simulink model "Capsuleuse_fermeture_geometrique"  (R2019b)
settings: Solver=VariableStepAuto  StartTime=0.0  StopTime=10.0  RelTol=1e-3
PreLoadFcn:
  | addpath('Simscape')
model workspace (MATLAB code in the model file):
  | % Simscape(TM) Multibody(TM) version: 7.0
  | 
  | % This is a model data file derived from a Simscape Multibody Import XML file using the smimport function.
  | % The data in this file sets the block parameter values in an imported Simscape Multibody model.
  | % For more information on this file, see the smimport function help page in the Simscape Multibody documentation.
  | % You can modify numerical values, but avoid any other changes to this file.
  | % Do not add code to this file. Do not edit the physical units shown in comments.
  | 
  | %%%VariableName:smiData
  | 
  | 
  | %============= RigidTransform =============%
  | 
  | %Initialize the RigidTransform structure array by filling in null values.
  | smiData.RigidTransform(76).translation = [0.0 0.0 0.0];
  | smiData.RigidTransform(76).angle = 0.0;
  | smiData.RigidTransform(76).axis = [0.0 0.0 0.0];
  | smiData.RigidTransform(76).ID = '';
  | 
  | %Translation Method - Cartesian
  | %Rotation Method - Arbitrary Axis
  | smiData.RigidTransform(1).translation = [0 0 0];  % mm
  | smiData.RigidTransform(1).angle = 2.2204460492503136e-16;  % rad
  | smiData.RigidTransform(1).axis = [-1 0 -0];
  | smiData.RigidTransform(1).ID = 'B[Bati-1:-:]';
  | 
  | %Translation Method - Cartesian
  | %Rotation Method - Arbitrary Axis
  | smiData.RigidTransform(2).translation = [0 0 0];  % mm
  | smiData.RigidTransform(2).angle = 3.1415926535897931;  % rad
  | smiData.RigidTransform(2).axis = [0 -1 -5.5511151231257839e-17];
  | smiData.RigidTransform(2).ID = 'F[Bati-1:-:]';
  | 
  | %Translation Method - Cartesian
  | %Rotation Method - Arbitrary Axis
  | smiData.RigidTransform(3).translation = [-1.4210854715202004e-14 8.8817841970012523e-14 125];  % mm
  | smiData.RigidTransform(3).angle = 2.0943951023931953;  % rad
  | smiData.RigidTransform(3).axis = [-0.57735026918962584 -0.57735026918962584 -0.57735026918962584];
  | smiData.RigidTransform(3).ID = 'B[Bati-1:-:Croix_de_Malte-1]';
  | 
  | %Translation Method - Cartesian
  | %Rotation Method - Arbitrary Axis
  | smiData.RigidTransform(4).translation = [1.8690460720473507e-12 22.000000000000014 -2.2892209790695388e-28];  % mm
  | smiData.RigidTransform(4).angle = 2.0943951023931953;  % rad
  | smiData.RigidTransform(4).axis = [-0.57735026918962584 -0.57735026918962562 -0.57735026918962595];
  | smiData.RigidTransform(4).ID = 'F[Bati-1:-:Croix_de_Malte-1]';
  | 
  | %Translation Method - Cartesian
  | %Rotation Method - Arbitrary Axis
  | smiData.RigidTransform(5).translation = [0 4.6185277824406512e-14 -3.5527136788005009e-15];  % mm
  | smiData.RigidTransform(5).angle = 2.0943951023931953;  % rad
  | smiData.RigidTransform(5).axis = [-0.57735026918962584 -0.57735026918962584 -0.57735026918962584];
  | smiData.RigidTransform(5).ID = 'B[Bati-1:-:Moteur-1]';
  | 
  | %Translation Method - Cartesian
  | %Rotation Method - Arbitrary Axis
  | smiData.RigidTransform(6).translation = [2.3777209295873426e-14 24.999999999999876 -3.6840445277123552e-15];  % mm
  | smiData.RigidTransform(6).angle = 2.0943951023931962;  % rad
  | smiData.RigidTransform(6).axis = [-0.57735026918962595 -0.57735026918962529 -0.57735026918962606];
  | smiData.RigidTransform(6).ID = 'F[Bati-1:-:Moteur-1]';
  | 
  | %Translation Method - Cartesian
  | %Rotation Method - Arbitrary Axis
  | smiData.RigidTransform(7).translation = [-18.73832970144344 11 -32.173358543987945];  % mm
  | smiData.RigidTransform(7).angle = 1.7177715174584023;  % rad
  | smiData.RigidTransform(7).axis = [-0.35740674433659403 -0.35740674433659386 0.86285620946101627];
  | smiData.RigidTransform(7).ID = 'B[Croix_de_Malte-1:-:rouleau galet-1]';
  | 
  | %Translation Method - Cartesian
  | %Rotation Method - Arbitrary Axis
  | smiData.RigidTransform(8).translation = [29.594858329028312 1.0000000000000657 -43.752922275812764];  % mm
  | smiData.RigidTransform(8).angle = 1.7206562415507236;  % rad
  | smiData.RigidTransform(8).axis = [0.36042318328087997 0.36042318328088008 0.86034310475958042];
  | smiData.RigidTransform(8).ID = 'F[Croix_de_Malte-1:-:rouleau galet-1]';
  | 
  | %Translation Method - Cartesian
  | %Rotation Method - Arbitrary Axis
  | smiData.RigidTransform(9).translation = [0 12.574722564734881 -0.13414733414733593];  % mm
  | smiData.RigidTransform(9).angle = 2.0943951023931953;  % rad
  | smiData.RigidTransform(9).axis = [-0.57735026918962584 -0.57735026918962584 -0.57735026918962584];
  | smiData.RigidTransform(9).ID = 'B[rouleau galet-1:-:Moteur-1]';
  | 
  | %Translation Method - Cartesian
  | %Rotation Method - Arbitrary Axis
  | smiData.RigidTransform(10).translation = [-4.2632564145606011e-14 25.574722564734707 88.390000000000057];  % mm
  | smiData.RigidTransform(10).angle = 2.0943951023931966;  % rad
  | smiData.RigidTransform(10).axis = [-0.57735026918962606 -0.5773502691896254 -0.57735026918962573];
  | smiData.RigidTransform(10).ID = 'F[rouleau galet-1:-:Moteur-1]';
  | 
  | %Translation Method - Cartesian
  | %Rotation Method - Arbitrary Axis
  | smiData.RigidTransform(11).translation = [-0.35889856916805629 20.000000000000071 84.999999999999986];  % mm
  | smiData.RigidTransform(11).angle = 3.1415926535897931;  % rad
  | smiData.RigidTransform(11).axis = [0 -0.70710678118654746 0.70710678118654757];
  | smiData.RigidTransform(11).ID = 'AssemblyGround[Bati-1:vis M6x20-2]';
  | 
  | %Translation Method - Cartesian
  | %Rotation Method - Arbitrary Axis
  | smiData.RigidTransform(12).translation = [0 7.0000000000000862 125];  % mm
  | smiData.RigidTransform(12).angle = 2.0943951023931957;  % rad
  | smiData.RigidTransform(12).axis = [-0.57735026918962562 -0.57735026918962562 0.57735026918962595];
  | smiData.RigidTransform(12).ID = 'AssemblyGround[Bati-1:boitier-1]';
  | 
  | %Translation Method - Cartesian
  | %Rotation Method - Arbitrary Axis
  | smiData.RigidTransform(13).translation = [69.999999999999986 12.000000000000032 -30.000000000000025];  % mm
  | smiData.RigidTransform(13).angle = 3.1415926535897931;  % rad
  | smiData.RigidTransform(13).axis = [0 -0.70710678118654746 0.70710678118654757];
  | smiData.RigidTransform(13).ID = 'AssemblyGround[Bati-1:plaque de base-1]';
  | 
  | %Translation Method - Cartesian
  | %Rotation Method - Arbitrary Axis
  | smiData.RigidTransform(14).translation = [39.999999999999993 20.000000000000089 125];  % mm
  | smiData.RigidTransform(14).angle = 3.1415926535897931;  % rad
  | smiData.RigidTransform(14).axis = [0 -0.70710678118654746 0.70710678118654757];
  | smiData.RigidTransform(14).ID = 'AssemblyGround[Bati-1:vis M6x20-1]';
  | 
  | %Translation Method - Cartesian
  | %Rotation Method - Arbitrary Axis
  | smiData.RigidTransform(15).translation = [194.99999999999994 25.000000000000124 235];  % mm
  | smiData.RigidTransform(15).angle = 3.1415926535897931;  % rad
  | smiData.RigidTransform(15).axis = [0 -0.70710678118654746 0.70710678118654757];
  | smiData.RigidTransform(15).ID = 'AssemblyGround[Bati-1:vis M8x25-2]';
  | 
  | %Translation Method - Cartesian
  | %Rotation Method - Arbitrary Axis
  | smiData.RigidTransform(16).translation = [-120.00000000000001 25.000000000000021 -55.000000000000043];  % mm
  | smiData.RigidTransform(16).angle = 3.1415926535897931;  % rad
  | smiData.RigidTransform(16).axis = [0 -0.70710678118654746 0.70710678118654757];
  | smiData.RigidTransform(16).ID = 'AssemblyGround[Bati-1:vis M8x25-3]';
  | 
  | %Translation Method - Cartesian
  | %Rotation Method - Arbitrary Axis
  | smiData.RigidTransform(17).translation = [194.99999999999994 25.00000000000006 39.999999999999986];  % mm
  | smiData.RigidTransform(17).angle = 3.1415926535897931;  % rad
  | smiData.RigidTransform(17).axis = [0 -0.70710678118654746 0.70710678118654757];
  | smiData.RigidTransform(17).ID = 'AssemblyGround[Bati-1:vis M8x25-1]';
  | 
  | %Translation Method - Cartesian
  | %Rotation Method - Arbitrary Axis
  | smiData.RigidTransform(18).translation = [-0.35889856916804241 20.000000000000099 165];  % mm
  | smiData.RigidTransform(18).angle = 3.1415926535897931;  % rad
  | smiData.RigidTransform(18).axis = [0 -0.70710678118654746 0.70710678118654757];
  | smiData.RigidTransform(18).ID = 'AssemblyGround[Bati-1:vis M6x20-3]';
  | 
  | %Translation Method - Cartesian
  | %Rotation Method - Arbitrary Axis
  | smiData.RigidTransform(19).translation = [-10.999999999999829 224.64380550980667 146.35619449019265];  % mm
  | smiData.RigidTransform(19).angle = 3.1415926535897833;  % rad
  | smiData.RigidTransform(19).axis = [0.70710678118654768 -2.3482086884408253e-15 0.70710678118654735];
  | smiData.RigidTransform(19).ID = 'AssemblyGround[Bati-1:rampe-1]';
  | 
  | %Translation Method - Cartesian
  | %Rotation Method - Arbitrary Axis
  | smiData.RigidTransform(20).translation = [-120.00000000000006 296.00000000000006 -54.999999999999929];  % mm
  | smiData.RigidTransform(20).angle = 1.6089415660457551;  % rad
  | smiData.RigidTransform(20).axis = [-0.96256421976262596 -0.19166392831303336 -0.19166392831303336];
  | smiData.RigidTransform(20).ID = 'AssemblyGround[Bati-1:vis M8x20-3]';
  | 
  | %Translation Method - Cartesian
  | %Rotation Method - Arbitrary Axis
  | smiData.RigidTransform(21).translation = [-109.00000000000003 310 -44.000000000000028];  % mm
  | smiData.RigidTransform(21).angle = 3.1415926535897931;  % rad
  | smiData.RigidTransform(21).axis = [0 -0.70710678118654746 0.70710678118654757];
  | smiData.RigidTransform(21).ID = 'AssemblyGround[Bati-1:pied-3]';
  | 
  | %Translation Method - Cartesian
  | %Rotation Method - Arbitrary Axis
  | smiData.RigidTransform(22).translation = [0 1.9999999999999658 -42.499999999999986];  % mm
  | smiData.RigidTransform(22).angle = 1.6654317068748059;  % rad
  | smiData.RigidTransform(22).axis = [-0.90957578911615289 -0.29382978393427672 -0.29382978393427672];
  | smiData.RigidTransform(22).ID = 'AssemblyGround[Bati-1:vis M6x20-6]';
  | 
  | %Translation Method - Cartesian
  | %Rotation Method - Arbitrary Axis
  | smiData.RigidTransform(23).translation = [205.99999999999997 310.00000000000011 246];  % mm
  | smiData.RigidTransform(23).angle = 3.1415926535897931;  % rad
  | smiData.RigidTransform(23).axis = [0 -0.70710678118654746 0.70710678118654757];
  | smiData.RigidTransform(23).ID = 'AssemblyGround[Bati-1:pied-1]';
  | 
  | %Translation Method - Cartesian
  | %Rotation Method - Arbitrary Axis
  | smiData.RigidTransform(24).translation = [194.99999999999994 296.00000000000011 235.00000000000003];  % mm
  | smiData.RigidTransform(24).angle = 1.6089415660457551;  % rad
  | smiData.RigidTransform(24).axis = [-0.96256421976262596 -0.19166392831303336 -0.19166392831303336];
  | smiData.RigidTransform(24).ID = 'AssemblyGround[Bati-1:vis M8x20-2]';
  | 
  | %Translation Method - Cartesian
  | %Rotation Method - Arbitrary Axis
  | smiData.RigidTransform(25).translation = [-32.000000000000071 185.00000000000009 418.00000000000006];  % mm
  | smiData.RigidTransform(25).angle = 1.5707963267948968;  % rad
  | smiData.RigidTransform(25).axis = [-1 2.081668171172168e-16 2.081668171172168e-16];
  | smiData.RigidTransform(25).ID = 'AssemblyGround[Bati-1:support-1]';
  | 
  | %Translation Method - Cartesian
  | %Rotation Method - Arbitrary Axis
  | smiData.RigidTransform(26).translation = [205.99999999999997 310.00000000000006 51.000000000000028];  % mm
  | smiData.RigidTransform(26).angle = 3.1415926535897931;  % rad
  | smiData.RigidTransform(26).axis = [0 -0.70710678118654746 0.70710678118654757];
  | smiData.RigidTransform(26).ID = 'AssemblyGround[Bati-1:pied-2]';
  | 
  | %Translation Method - Cartesian
  | %Rotation Method - Arbitrary Axis
  | smiData.RigidTransform(27).translation = [0 7.0000000000000409 0];  % mm
  | smiData.RigidTransform(27).angle = 3.1415926535897931;  % rad
  | smiData.RigidTransform(27).axis = [0.70710678118654768 1.218024257459634e-16 0.70710678118654735];
  | smiData.RigidTransform(27).ID = 'AssemblyGround[Bati-1:motoreducteur-1]';
  | 
  | %Translation Method - Cartesian
  | %Rotation Method - Arbitrary Axis
  | smiData.RigidTransform(28).translation = [42.499999999999993 2.0000000000001523 0];  % mm
  | smiData.RigidTransform(28).angle = 1.7612805946572963;  % rad
  | smiData.RigidTransform(28).axis = [-0.82559845262457221 -0.39899072359135895 -0.39899072359135845];
  | smiData.RigidTransform(28).ID = 'AssemblyGround[Bati-1:vis M6x20-5]';
  | 
  | %Translation Method - Cartesian
  | %Rotation Method - Arbitrary Axis
  | smiData.RigidTransform(29).translation = [299.99999999999994 316.00000000000017 430];  % mm
  | smiData.RigidTransform(29).angle = 3.1415926535897931;  % rad
  | smiData.RigidTransform(29).axis = [0 -0.70710678118654746 0.70710678118654757];
  | smiData.RigidTransform(29).ID = 'AssemblyGround[Bati-1:bati-1]';
  | 
  | %Translation Method - Cartesian
  | %Rotation Method - Arbitrary Axis
  | smiData.RigidTransform(30).translation = [194.99999999999991 296.00000000000006 40.000000000000043];  % mm
  | smiData.RigidTransform(30).angle = 1.6089415660457551;  % rad
  | smiData.RigidTransform(30).axis = [-0.96256421976262596 -0.19166392831303336 -0.19166392831303336];
  | smiData.RigidTransform(30).ID = 'AssemblyGround[Bati-1:vis M8x20-1]';
  | 
  | %Translation Method - Cartesian
  | %Rotation Method - Arbitrary Axis
  | smiData.RigidTransform(31).translation = [-40.000000000000007 20.000000000000089 125.00000000000003];  % mm
  | smiData.RigidTransform(31).angle = 3.1415926535897931;  % rad
  | smiData.RigidTransform(31).axis = [0 -0.70710678118654746 0.70710678118654757];
  | smiData.RigidTransform(31).ID = 'AssemblyGround[Bati-1:vis M6x20-4]';
  | 
  | %Translation Method - Cartesian
  | %Rotation Method - Arbitrary Axis
  | smiData.RigidTransform(32).translation = [0 2.0000000000000751 42.500000000000007];  % mm
  | smiData.RigidTransform(32).angle = 1.6333821857835207;  % rad
  | smiData.RigidTransform(32).axis = [-0.9392939931105766 -0.24261780077561093 -0.24261780077561074];
  | smiData.RigidTransform(32).ID = 'AssemblyGround[Bati-1:vis M6x20-7]';
  | 
  | %Translation Method - Cartesian
  | %Rotation Method - Arbitrary Axis
  | smiData.RigidTransform(33).translation = [-42.500000000000007 2.000000000000107 0];  % mm
  | smiData.RigidTransform(33).angle = 1.7546548549139718;  % rad
  | smiData.RigidTransform(33).axis = [-0.83118471645013647 -0.3931488058863376 -0.39314880588633738];
  | smiData.RigidTransform(33).ID = 'AssemblyGround[Bati-1:vis M6x20-8]';
  | 
  | %Translation Method - Cartesian
  | %Rotation Method - Arbitrary Axis
  | smiData.RigidTransform(34).translation = [-35.355339059327292 213.50000000000003 -35.355339059327434];  % mm
  | smiData.RigidTransform(34).angle = 3.1415926535897909;  % rad
  | smiData.RigidTransform(34).axis = [1.2601194582917002e-15 0.70710678118654746 -0.70710678118654757];
  | smiData.RigidTransform(34).ID = 'AssemblyGround[Croix_de_Malte-1:ecrou M12-1]';
  | 
  | %Translation Method - Cartesian
  | %Rotation Method - Arbitrary Axis
  | smiData.RigidTransform(35).translation = [-15.999999999999963 16.999999999999996 6.9999999999999503];  % mm
  | smiData.RigidTransform(35).angle = 2.0943951023931953;  % rad
  | smiData.RigidTransform(35).axis = [0.57735026918962584 -0.57735026918962584 0.57735026918962584];
  | smiData.RigidTransform(35).ID = 'AssemblyGround[Croix_de_Malte-1:goupille D6-1]';
  | 
  | %Translation Method - Cartesian
  | %Rotation Method - Arbitrary Axis
  | smiData.RigidTransform(36).translation = [15.999999999999993 16.999999999999993 7.0000000000000338];  % mm
  | smiData.RigidTransform(36).angle = 3.0512029265937719;  % rad
  | smiData.RigidTransform(36).axis = [0.045225659969685389 0.70638326695934206 -0.70638326695934206];
  | smiData.RigidTransform(36).ID = 'AssemblyGround[Croix_de_Malte-1:goupille D6-2]';
  | 
  | %Translation Method - Cartesian
  | %Rotation Method - Arbitrary Axis
  | smiData.RigidTransform(37).translation = [0 180 0];  % mm
  | smiData.RigidTransform(37).angle = 1.5707963267948966;  % rad
  | smiData.RigidTransform(37).axis = [0 0 1];
  | smiData.RigidTransform(37).ID = 'AssemblyGround[Croix_de_Malte-1:bride-1]';
  | 
  | %Translation Method - Cartesian
  | %Rotation Method - Arbitrary Axis
  | smiData.RigidTransform(38).translation = [67.500000000000028 209.99999999999997 0];  % mm
  | smiData.RigidTransform(38).angle = 2.0943951023931953;  % rad
  | smiData.RigidTransform(38).axis = [0.57735026918962584 -0.57735026918962584 0.57735026918962584];
  | smiData.RigidTransform(38).ID = 'AssemblyGround[Croix_de_Malte-1:vis M6x30-2]';
  | 
  | %Translation Method - Cartesian
  | %Rotation Method - Arbitrary Axis
  | smiData.RigidTransform(39).translation = [0 221 0];  % mm
  | smiData.RigidTransform(39).angle = 3.1415926535897922;  % rad
  | smiData.RigidTransform(39).axis = [6.713347862852846e-16 0.70710678118654746 -0.70710678118654757];
  | smiData.RigidTransform(39).ID = 'AssemblyGround[Croix_de_Malte-1:plateau-1]';
  | 
  | %Translation Method - Cartesian
  | %Rotation Method - Arbitrary Axis
  | smiData.RigidTransform(40).translation = [0 210 -67.5];  % mm
  | smiData.RigidTransform(40).angle = 2.0943951023931953;  % rad
  | smiData.RigidTransform(40).axis = [0.57735026918962584 -0.57735026918962584 0.57735026918962584];
  | smiData.RigidTransform(40).ID = 'AssemblyGround[Croix_de_Malte-1:vis M6x30-4]';
  | 
  | %Translation Method - Cartesian
  | %Rotation Method - Arbitrary Axis
  | smiData.RigidTransform(41).translation = [-35.355339059327292 195 -35.355339059327434];  % mm
  | smiData.RigidTransform(41).angle = 1.5744668381809315;  % rad
  | smiData.RigidTransform(41).axis = [-0.9963362084947659 0.060473794499247502 0.06047379449924746];
  | smiData.RigidTransform(41).ID = 'AssemblyGround[Croix_de_Malte-1:vis a billes-1]';
  | 
  | %Translation Method - Cartesian
  | %Rotation Method - Arbitrary Axis
  | smiData.RigidTransform(42).translation = [0 145 0];  % mm
  | smiData.RigidTransform(42).angle = 1.7177715174584023;  % rad
  | smiData.RigidTransform(42).axis = [-0.35740674433659392 -0.35740674433659392 0.86285620946101627];
  | smiData.RigidTransform(42).ID = 'AssemblyGround[Croix_de_Malte-1:limiteur couple-1]';
  | 
  | %Translation Method - Cartesian
  | %Rotation Method - Arbitrary Axis
  | smiData.RigidTransform(43).translation = [0 159.99999999999994 -22.500000000000007];  % mm
  | smiData.RigidTransform(43).angle = 1.8369463418012444;  % rad
  | smiData.RigidTransform(43).axis = [-3.8857805861880479e-16 -3.0765813436776594e-16 1];
  | smiData.RigidTransform(43).ID = 'AssemblyGround[Croix_de_Malte-1:mecanindus-1]';
  | 
  | %Translation Method - Cartesian
  | %Rotation Method - Arbitrary Axis
  | smiData.RigidTransform(44).translation = [0 210.00000000000003 67.5];  % mm
  | smiData.RigidTransform(44).angle = 2.0943951023931953;  % rad
  | smiData.RigidTransform(44).axis = [0.57735026918962584 -0.57735026918962584 0.57735026918962584];
  | smiData.RigidTransform(44).ID = 'AssemblyGround[Croix_de_Malte-1:vis M6x30-1]';
  | 
  | %Translation Method - Cartesian
  | %Rotation Method - Arbitrary Axis
  | smiData.RigidTransform(45).translation = [-67.499999999999972 210 0];  % mm
  | smiData.RigidTransform(45).angle = 2.0943951023931953;  % rad
  | smiData.RigidTransform(45).axis = [0.57735026918962584 -0.57735026918962584 0.57735026918962584];
  | smiData.RigidTransform(45).ID = 'AssemblyGround[Croix_de_Malte-1:vis M6x30-3]';
  | 
  | %Translation Method - Cartesian
  | %Rotation Method - Arbitrary Axis
  | smiData.RigidTransform(46).translation = [0 0 0];  % mm
  | smiData.RigidTransform(46).angle = 0;  % rad
  | smiData.RigidTransform(46).axis = [0 0 0];
  | smiData.RigidTransform(46).ID = 'AssemblyGround[Croix_de_Malte-1:6004-2:BI 6004-1]';
  | 
  | %Translation Method - Cartesian
  | %Rotation Method - Arbitrary Axis
  | smiData.RigidTransform(47).translation = [0 0 0];  % mm
  | smiData.RigidTransform(47).angle = 0;  % rad
  | smiData.RigidTransform(47).axis = [0 0 0];
  | smiData.RigidTransform(47).ID = 'AssemblyGround[Croix_de_Malte-1:6004-2:bille 6004-1]';
  | 
  | %Translation Method - Cartesian
  | %Rotation Method - Arbitrary Axis
  | smiData.RigidTransform(48).translation = [0 0 0];  % mm
  | smiData.RigidTransform(48).angle = 0;  % rad
  | smiData.RigidTransform(48).axis = [0 0 0];
  | smiData.RigidTransform(48).ID = 'AssemblyGround[Croix_de_Malte-1:6004-2:BE 6004-1]';
  | 
  | %Translation Method - Cartesian
  | %Rotation Method - Arbitrary Axis
  | smiData.RigidTransform(49).translation = [87.500000000000014 134 0];  % mm
  | smiData.RigidTransform(49).angle = 1.5707963267948966;  % rad
  | smiData.RigidTransform(49).axis = [0 0 1];
  | smiData.RigidTransform(49).ID = 'AssemblyGround[Croix_de_Malte-1:6004-2]';
  | 
  | %Translation Method - Cartesian
  | %Rotation Method - Arbitrary Axis
  | smiData.RigidTransform(50).translation = [0 -19 49.999999999999986];  % mm
  | smiData.RigidTransform(50).angle = 1.5707963267948966;  % rad
  | smiData.RigidTransform(50).axis = [0 0 1];
  | smiData.RigidTransform(50).ID = 'AssemblyGround[Croix_de_Malte-1:doigt-1]';
  | 
  | %Translation Method - Cartesian
  | %Rotation Method - Arbitrary Axis
  | smiData.RigidTransform(51).translation = [0 -1.0000000000000009 0];  % mm
  | smiData.RigidTransform(51).angle = 1.5707963267948966;  % rad
  | smiData.RigidTransform(51).axis = [0 0 1];
  | smiData.RigidTransform(51).ID = 'AssemblyGround[Croix_de_Malte-1:axe de sortie-1]';
  | 
  | %Translation Method - Cartesian
  | %Rotation Method - Arbitrary Axis
  | smiData.RigidTransform(52).translation = [0 0 0];  % mm
  | smiData.RigidTransform(52).angle = 2.0943951023931966;  % rad
  | smiData.RigidTransform(52).axis = [-0.57735026918962618 -0.57735026918962606 0.57735026918962495];
  | smiData.RigidTransform(52).ID = 'AssemblyGround[Croix_de_Malte-1:croix-1]';
  | 
  | %Translation Method - Cartesian
  | %Rotation Method - Arbitrary Axis
  | smiData.RigidTransform(53).translation = [0 -1.0000000000000009 0];  % mm
  | smiData.RigidTransform(53).angle = 2.0943951023931966;  % rad
  | smiData.RigidTransform(53).axis = [0.57735026918962495 -0.57735026918962618 0.57735026918962618];
  | smiData.RigidTransform(53).ID = 'AssemblyGround[Croix_de_Malte-1:capteur-1]';
  | 
  | %Translation Method - Cartesian
  | %Rotation Method - Arbitrary Axis
  | smiData.RigidTransform(54).translation = [0 11.999999999999998 16.000000000000014];  % mm
  | smiData.RigidTransform(54).angle = 2.0943951023931953;  % rad
  | smiData.RigidTransform(54).axis = [0.57735026918962584 -0.57735026918962584 0.57735026918962584];
  | smiData.RigidTransform(54).ID = 'AssemblyGround[Croix_de_Malte-1:vis M6x25-1]';
  | 
  | %Translation Method - Cartesian
  | %Rotation Method - Arbitrary Axis
  | smiData.RigidTransform(55).translation = [0 0 0];  % mm
  | smiData.RigidTransform(55).angle = 0;  % rad
  | smiData.RigidTransform(55).axis = [0 0 0];
  | smiData.RigidTransform(55).ID = 'AssemblyGround[Croix_de_Malte-1:6004-1:BI 6004-1]';
  | 
  | %Translation Method - Cartesian
  | %Rotation Method - Arbitrary Axis
  | smiData.RigidTransform(56).translation = [0 0 0];  % mm
  | smiData.RigidTransform(56).angle = 0;  % rad
  | smiData.RigidTransform(56).axis = [0 0 0];
  | smiData.RigidTransform(56).ID = 'AssemblyGround[Croix_de_Malte-1:6004-1:bille 6004-1]';
  | 
  | %Translation Method - Cartesian
  | %Rotation Method - Arbitrary Axis
  | smiData.RigidTransform(57).translation = [0 0 0];  % mm
  | smiData.RigidTransform(57).angle = 0;  % rad
  | smiData.RigidTransform(57).axis = [0 0 0];
  | smiData.RigidTransform(57).ID = 'AssemblyGround[Croix_de_Malte-1:6004-1:BE 6004-1]';
  | 
  | %Translation Method - Cartesian
  | %Rotation Method - Arbitrary Axis
  | smiData.RigidTransform(58).translation = [87.500000000000014 55.999999999999979 0];  % mm
  | smiData.RigidTransform(58).angle = 1.5707963267948966;  % rad
  | smiData.RigidTransform(58).axis = [0 0 1];
  | smiData.RigidTransform(58).ID = 'AssemblyGround[Croix_de_Malte-1:6004-1]';
  | 
  | %Translation Method - Cartesian
  | %Rotation Method - Arbitrary Axis
  | smiData.RigidTransform(59).translation = [0 -12.000000000000004 0];  % mm
  | smiData.RigidTransform(59).angle = 2.0943951023931948;  % rad
  | smiData.RigidTransform(59).axis = [0.57735026918962629 0.57735026918962562 0.57735026918962551];
  | smiData.RigidTransform(59).ID = 'AssemblyGround[Moteur-1:indexeur-1]';
  | 
  | %Translation Method - Cartesian
  | %Rotation Method - Arbitrary Axis
  | smiData.RigidTransform(60).translation = [0 -24.000000000000007 0];  % mm
  | smiData.RigidTransform(60).angle = 2.0943951023931953;  % rad
  | smiData.RigidTransform(60).axis = [-0.57735026918962584 0.57735026918962584 0.57735026918962584];
  | smiData.RigidTransform(60).ID = 'AssemblyGround[Moteur-1:capteur-1]';
  | 
  | %Translation Method - Cartesian
  | %Rotation Method - Arbitrary Axis
  | smiData.RigidTransform(61).translation = [0 -20.499999999999886 88.390000000000001];  % mm
  | smiData.RigidTransform(61).angle = 1.6445462178112022;  % rad
  | smiData.RigidTransform(61).axis = [-0.9288418077937356 0.26196650176545955 0.26196650176545944];
  | smiData.RigidTransform(61).ID = 'AssemblyGround[Moteur-1:ecrou M8-1]';
  | 
  | %Translation Method - Cartesian
  | %Rotation Method - Arbitrary Axis
  | smiData.RigidTransform(62).translation = [0 -13.000000000000005 0];  % mm
  | smiData.RigidTransform(62).angle = 2.0943951023931948;  % rad
  | smiData.RigidTransform(62).axis = [-0.57735026918962618 -0.57735026918962551 0.57735026918962562];
  | smiData.RigidTransform(62).ID = 'AssemblyGround[Moteur-1:arbre moteur-1]';
  | 
  | %Translation Method - Cartesian
  | %Rotation Method - Arbitrary Axis
  | smiData.RigidTransform(63).translation = [0 17 -35.000000000000007];  % mm
  | smiData.RigidTransform(63).angle = 2.0943951023931953;  % rad
  | smiData.RigidTransform(63).axis = [0.57735026918962573 0.57735026918962573 -0.57735026918962584];
  | smiData.RigidTransform(63).ID = 'AssemblyGround[Moteur-1:goupille D10-1]';
  | 
  | %Translation Method - Cartesian
  | %Rotation Method - Arbitrary Axis
  | smiData.RigidTransform(64).translation = [35 0 -35.000000000000014];  % mm
  | smiData.RigidTransform(64).angle = 2.0943951023931948;  % rad
  | smiData.RigidTransform(64).axis = [0.57735026918962562 -0.57735026918962618 0.57735026918962551];
  | smiData.RigidTransform(64).ID = 'AssemblyGround[Moteur-1:maneton-1]';
  | 
  | %Translation Method - Cartesian
  | %Rotation Method - Arbitrary Axis
  | smiData.RigidTransform(65).translation = [0 -30.000000000000021 -50.000000000000014];  % mm
  | smiData.RigidTransform(65).angle = 1.6401005108791142;  % rad
  | smiData.RigidTransform(65).axis = [0.25448752703143285 0.25448752703143285 0.93299099522495466];
  | smiData.RigidTransform(65).ID = 'AssemblyGround[Moteur-1:doigt-1]';
  | 
  | %Translation Method - Cartesian
  | %Rotation Method - Arbitrary Axis
  | smiData.RigidTransform(66).translation = [0 0 88.390000000000001];  % mm
  | smiData.RigidTransform(66).angle = 1.5707963267948966;  % rad
  | smiData.RigidTransform(66).axis = [0 0 1];
  | smiData.RigidTransform(66).ID = 'AssemblyGround[Moteur-1:rondelle galet-1]';
  | 
  | %Translation Method - Cartesian
  | %Rotation Method - Arbitrary Axis
  | smiData.RigidTransform(67).translation = [0 -14.000000000000005 88.390000000000015];  % mm
  | smiData.RigidTransform(67).angle = 1.5707963267948966;  % rad
  | smiData.RigidTransform(67).axis = [0 0 1];
  | smiData.RigidTransform(67).ID = 'AssemblyGround[Moteur-1:rondelle galet-2]';
  | 
  | %Translation Method - Cartesian
  | %Rotation Method - Arbitrary Axis
  | smiData.RigidTransform(68).translation = [0 11.99999999999989 88.390000000000015];  % mm
  | smiData.RigidTransform(68).angle = 2.3824818043914275;  % rad
  | smiData.RigidTransform(68).axis = [-0.64841380796894177 0.64841380796894188 -0.39889731419305452];
  | smiData.RigidTransform(68).ID = 'AssemblyGround[Moteur-1:axe galet-1]';
  | 
  | %Translation Method - Cartesian
  | %Rotation Method - Arbitrary Axis
  | smiData.RigidTransform(69).translation = [0 5.9999999999999876 -16.000000000000011];  % mm
  | smiData.RigidTransform(69).angle = 2.8654427051283657;  % rad
  | smiData.RigidTransform(69).axis = [0.13895917020031051 -0.70024650981537961 0.70024650981537961];
  | smiData.RigidTransform(69).ID = 'AssemblyGround[Moteur-1:vis M6x30-1]';
  | 
  | %Translation Method - Cartesian
  | %Rotation Method - Arbitrary Axis
  | smiData.RigidTransform(70).translation = [16.000000000000036 -24.000000000000014 -7.0000000000000107];  % mm
  | smiData.RigidTransform(70).angle = 2.0943951023931953;  % rad
  | smiData.RigidTransform(70).axis = [-0.57735026918962584 0.57735026918962584 0.57735026918962584];
  | smiData.RigidTransform(70).ID = 'AssemblyGround[Moteur-1:goupille D6-1]';
  | 
  | %Translation Method - Cartesian
  | %Rotation Method - Arbitrary Axis
  | smiData.RigidTransform(71).translation = [3.0000000000001505 143.00000000000006 -6.8543636114536088];  % mm
  | smiData.RigidTransform(71).angle = 3.1415926535897922;  % rad
  | smiData.RigidTransform(71).axis = [-3.3080175810533039e-16 -0.70710678118654746 0.70710678118654757];
  | smiData.RigidTransform(71).ID = 'AssemblyGround[Moteur-1:clavette-1]';
  | 
  | %Translation Method - Cartesian
  | %Rotation Method - Arbitrary Axis
  | smiData.RigidTransform(72).translation = [0.48219033392770183 152.99999999999991 0.1322591466277776];  % mm
  | smiData.RigidTransform(72).angle = 1.5886069344924167;  % rad
  | smiData.RigidTransform(72).axis = [-0.13228012687504107 -0.13228012687504107 0.98234613862316666];
  | smiData.RigidTransform(72).ID = 'AssemblyGround[Moteur-1:rondelle arbre moteur-1]';
  | 
  | %Translation Method - Cartesian
  | %Rotation Method - Arbitrary Axis
  | smiData.RigidTransform(73).translation = [-25.999999999999993 13.999999999999979 26.000000000000011];  % mm
  | smiData.RigidTransform(73).angle = 2.4027929767070448;  % rad
  | smiData.RigidTransform(73).axis = [0.38717287369613024 -0.65195750086715021 0.6519575008671501];
  | smiData.RigidTransform(73).ID = 'AssemblyGround[Moteur-1:vis M6x20-1]';
  | 
  | %Translation Method - Cartesian
  | %Rotation Method - Arbitrary Axis
  | smiData.RigidTransform(74).translation = [0 142.00000000000003 0];  % mm
  | smiData.RigidTransform(74).angle = 2.0190968955024911;  % rad
  | smiData.RigidTransform(74).axis = [-0.62868927457125068 0.54988625916596368 0.54988625916596356];
  | smiData.RigidTransform(74).ID = 'AssemblyGround[Moteur-1:vis M6x15-1]';
  | 
  | %Translation Method - Cartesian
  | %Rotation Method - Arbitrary Axis
  | smiData.RigidTransform(75).translation = [-15.999999999999979 -24 -7.0000000000000071];  % mm
  | smiData.RigidTransform(75).angle = 2.0943951023931953;  % rad
  | smiData.RigidTransform(75).axis = [-0.57735026918962584 0.57735026918962584 0.57735026918962584];
  | smiData.RigidTransform(75).ID = 'AssemblyGround[Moteur-1:goupille D6-2]';
  | 
  | %Translation Method - Cartesian
  | %Rotation Method - Arbitrary Axis
  | smiData.RigidTransform(76).translation = [26.000000000000007 14.000000000000021 -26.000000000000014];  % mm
  | smiData.RigidTransform(76).angle = 3.1185481265020982;  % rad
  | smiData.RigidTransform(76).axis = [0.011522773479318524 0.70705983682123552 -0.70705983682123552];
  | smiData.RigidTransform(76).ID = 'AssemblyGround[Moteur-1:vis M6x20-2]';
  | 
  | 
  | %============= Solid =============%
  | %Center of Mass (CoM) %Moments of Inertia (MoI) %Product of Inertia (PoI)
  | 
  | %Initialize the Solid structure array by filling in null values.
  | smiData.Solid(37).mass = 0.0;
  | smiData.Solid(37).CoM = [0.0 0.0 0.0];
  | smiData.Solid(37).MoI = [0.0 0.0 0.0];
  | smiData.Solid(37).PoI = [0.0 0.0 0.0];
  | smiData.Solid(37).color = [0.0 0.0 0.0];
  | smiData.Solid(37).opacity = 0.0;
  | smiData.Solid(37).ID = '';
  | 
  | %Inertia Type - Custom
  | %Visual Properties - Simple
  | smiData.Solid(1).mass = 0.00097601953307612085;  % kg
  | smiData.Solid(1).CoM = [0 0 15.44244610393042];  % mm
  | smiData.Solid(1).MoI = [0.06287794871934245 0.06287794871934245 0.0082297985935085305];  % kg*mm^2
  | smiData.Solid(1).PoI = [0 0 0];  % kg*mm^2
  | smiData.Solid(1).color = [0.792156862745098 0.81960784313725488 0.93333333333333335];
  | smiData.Solid(1).opacity = 1;
  | smiData.Solid(1).ID = 'vis M6x20*:*Defaut';
  | 
  | %Inertia Type - Custom
  | %Visual Properties - Simple
  | smiData.Solid(2).mass = 0.1943668817256817;  % kg
  | smiData.Solid(2).CoM = [46.229215324662299 0 0];  % mm
  | smiData.Solid(2).MoI = [160.45640918614012 301.04291141244755 301.04291141244755];  % kg*mm^2
  | smiData.Solid(2).PoI = [0 0 0];  % kg*mm^2
  | smiData.Solid(2).color = [0 0.50196078431372548 1];
  | smiData.Solid(2).opacity = 0.73999999999999999;
  | smiData.Solid(2).ID = 'boitier*:*Defaut';
  | 
  | %Inertia Type - Custom
  | %Visual Properties - Simple
  | smiData.Solid(3).mass = 1.2084987927862845;  % kg
  | smiData.Solid(3).CoM = [29.061310422302391 -121.73973572259008 6.0932460832211488];  % mm
  | smiData.Solid(3).MoI = [10469.336534607892 12874.507918055215 23315.399325681959];  % kg*mm^2
  | smiData.Solid(3).PoI = [-1.4552932788796373 -4.6128131769759255 113.51826268485617];  % kg*mm^2
  | smiData.Solid(3).color = [1 1 0];
  | smiData.Solid(3).opacity = 0.75;
  | smiData.Solid(3).ID = 'plaque de base*:*Defaut';
  | 
  | %Inertia Type - Custom
  | %Visual Properties - Simple
  | smiData.Solid(4).mass = 0.0022042120101588864;  % kg
  | smiData.Solid(4).CoM = [0 0 19.517428266608167];  % mm
  | smiData.Solid(4).MoI = [0.22773602672305743 0.22773602672305743 0.031806951209625595];  % kg*mm^2
  | smiData.Solid(4).PoI = [0 0 0];  % kg*mm^2
  | smiData.Solid(4).color = [0.75294117647058822 0.75294117647058822 0.75294117647058822];
  | smiData.Solid(4).opacity = 1;
  | smiData.Solid(4).ID = 'vis M8x25*:*Defaut';
  | 
  | %Inertia Type - Custom
  | %Visual Properties - Simple
  | smiData.Solid(5).mass = 0.21286544470158805;  % kg
  | smiData.Solid(5).CoM = [94.029303331746007 -0.82762910036634985 -3.735221012653803e-06];  % mm
  | smiData.Solid(5).MoI = [2338.7918105424051 3452.5238460592213 1172.7207081207969];  % kg*mm^2
  | smiData.Solid(5).PoI = [-2.7113766148496268e-05 9.5684464676638341e-05 -84.870049303396272];  % kg*mm^2
  | smiData.Solid(5).color = [0.50196078431372548 1 0.50196078431372548];
  | smiData.Solid(5).opacity = 1;
  | smiData.Solid(5).ID = 'rampe*:*Defaut';
  | 
  | %Inertia Type - Custom
  | %Visual Properties - Simple
  | smiData.Solid(6).mass = 0.0019528845978717027;  % kg
  | smiData.Solid(6).CoM = [0 0 16.699785969605902];  % mm
  | smiData.Solid(6).MoI = [0.14463078865869303 0.14463078865869303 0.029796331911328133];  % kg*mm^2
  | smiData.Solid(6).PoI = [0 0 0];  % kg*mm^2
  | smiData.Solid(6).color = [0.75294117647058822 0.75294117647058822 0.75294117647058822];
  | smiData.Solid(6).opacity = 1;
  | smiData.Solid(6).ID = 'vis M8x20*:*Defaut';
  | 
  | %Inertia Type - Custom
  | %Visual Properties - Simple
  | smiData.Solid(7).mass = 0.14244276480901016;  % kg
  | smiData.Solid(7).CoM = [10.999999999999998 10.999999999999998 149];  % mm
  | smiData.Solid(7).MoI = [1039.7464728197081 1039.7464728197081 11.62452441311798];  % kg*mm^2
  | smiData.Solid(7).PoI = [0 0 0];  % kg*mm^2
  | smiData.Solid(7).color = [0.75294117647058822 0.75294117647058822 0.75294117647058822];
  | smiData.Solid(7).opacity = 1;
  | smiData.Solid(7).ID = 'pied*:*Defaut';
  | 
  | %Inertia Type - Custom
  | %Visual Properties - Simple
  | smiData.Solid(8).mass = 0.10055611901672681;  % kg
  | smiData.Solid(8).CoM = [21 10.000000000000002 62.705915274303955];  % mm
  | smiData.Solid(8).MoI = [130.65443989906203 142.13320856911679 18.2916020303539];  % kg*mm^2
  | smiData.Solid(8).PoI = [0 0 0];  % kg*mm^2
  | smiData.Solid(8).color = [1 0.50196078431372548 0];
  | smiData.Solid(8).opacity = 1;
  | smiData.Solid(8).ID = 'support*:*Defaut';
  | 
  | %Inertia Type - Custom
  | %Visual Properties - Simple
  | smiData.Solid(9).mass = 2.4806817318400451;  % kg
  | smiData.Solid(9).CoM = [-32.469794728886221 -77.614477112305821 96.552435724812568];  % mm
  | smiData.Solid(9).MoI = [21244.763105758535 21718.212100504341 3934.2344587272351];  % kg*mm^2
  | smiData.Solid(9).PoI = [571.37057426684703 1803.6036175960992 -192.14725264359842];  % kg*mm^2
  | smiData.Solid(9).color = [1 0.50196078431372548 0.50196078431372548];
  | smiData.Solid(9).opacity = 0.75;
  | smiData.Solid(9).ID = 'motoreducteur*:*Defaut';
  | 
  | %Inertia Type - Custom
  | %Visual Properties - Simple
  | smiData.Solid(10).mass = 2.0265803928196586;  % kg
  | smiData.Solid(10).CoM = [260.01517949910749 325.04357537046548 3];  % mm
  | smiData.Solid(10).MoI = [71356.103707353715 45677.514095400678 117021.45832039748];  % kg*mm^2
  | smiData.Solid(10).PoI = [0 0 5.9942752262732384];  % kg*mm^2
  | smiData.Solid(10).color = [0.50196078431372548 1 1];
  | smiData.Solid(10).opacity = 1;
  | smiData.Solid(10).ID = 'bati*:*Defaut';
  | 
  | %Inertia Type - Custom
  | %Visual Properties - Simple
  | smiData.Solid(11).mass = 0.0012321195738996355;  % kg
  | smiData.Solid(11).CoM = [-3.6681762461281119e-07 0.00034962742306409188 3.2500000034909218];  % mm
  | smiData.Solid(11).MoI = [0.040028429648495102 0.040029009436780207 0.071591311827002707];  % kg*mm^2
  | smiData.Solid(11).PoI = [-8.482444639847799e-08 0 0];  % kg*mm^2
  | smiData.Solid(11).color = [1 0.50196078431372548 0.50196078431372548];
  | smiData.Solid(11).opacity = 1;
  | smiData.Solid(11).ID = 'ecrou M12*:*Defaut';
  | 
  | %Inertia Type - Custom
  | %Visual Properties - Simple
  | smiData.Solid(12).mass = 0.0008437794268766586;  % kg
  | smiData.Solid(12).CoM = [0 0 14.999999999999998];  % mm
  | smiData.Solid(12).MoI = [0.064528820341048204 0.064528820341048204 0.003781122743090253];  % kg*mm^2
  | smiData.Solid(12).PoI = [0 0 0];  % kg*mm^2
  | smiData.Solid(12).color = [1 0.50196078431372548 0];
  | smiData.Solid(12).opacity = 1;
  | smiData.Solid(12).ID = 'goupille D6*:*Defaut';
  | 
  | %Inertia Type - Custom
  | %Visual Properties - Simple
  | smiData.Solid(13).mass = 0.10662675422026636;  % kg
  | smiData.Solid(13).CoM = [6.878505230499977 0 0];  % mm
  | smiData.Solid(13).MoI = [472.9095682055995 238.52329716439436 238.52329716439436];  % kg*mm^2
  | smiData.Solid(13).PoI = [0 0 0];  % kg*mm^2
  | smiData.Solid(13).color = [0.75294117647058822 0.75294117647058822 0.75294117647058822];
  | smiData.Solid(13).opacity = 1;
  | smiData.Solid(13).ID = 'bride*:*Defaut';
  | 
  | %Inertia Type - Custom
  | %Visual Properties - Simple
  | smiData.Solid(14).mass = 0.0012587628718992024;  % kg
  | smiData.Solid(14).CoM = [0 0 20.868341921395942];  % mm
  | smiData.Solid(14).MoI = [0.1567882886725066 0.1567882886725066 0.0095021436182123904];  % kg*mm^2
  | smiData.Solid(14).PoI = [0 0 0];  % kg*mm^2
  | smiData.Solid(14).color = [0.792156862745098 0.81960784313725488 0.93333333333333335];
  | smiData.Solid(14).opacity = 1;
  | smiData.Solid(14).ID = 'vis M6x30*:*Defaut';
  | 
  | %Inertia Type - Custom
  | %Visual Properties - Simple
  | smiData.Solid(15).mass = 2.6954697137883201;  % kg
  | smiData.Solid(15).CoM = [-0.2047161049877978 -0.20471610498783416 13.028195979753319];  % mm
  | smiData.Solid(15).MoI = [24477.099012565133 24477.099012565141 48650.411388032553];  % kg*mm^2
  | smiData.Solid(15).PoI = [-2.7026143135195508 -2.7026143135196903 19.622253966311845];  % kg*mm^2
  | smiData.Solid(15).color = [0.75294117647058822 0.75294117647058822 0.75294117647058822];
  | smiData.Solid(15).opacity = 1;
  | smiData.Solid(15).ID = 'plateau*:*Defaut';
  | 
  | %Inertia Type - Custom
  | %Visual Properties - Simple
  | smiData.Solid(16).mass = 0.0023271645312013894;  % kg
  | smiData.Solid(16).CoM = [0 0 9.3805920598193389];  % mm
  | smiData.Solid(16).MoI = [0.10472373328422112 0.10499213692777545 0.040427824749548195];  % kg*mm^2
  | smiData.Solid(16).PoI = [0 0 0];  % kg*mm^2
  | smiData.Solid(16).color = [0.50196078431372548 0.50196078431372548 1];
  | smiData.Solid(16).opacity = 1;
  | smiData.Solid(16).ID = 'vis a billes*:*Defaut';
  | 
  | %Inertia Type - Custom
  | %Visual Properties - Simple
  | smiData.Solid(17).mass = 0.17170849125984147;  % kg
  | smiData.Solid(17).CoM = [37.92038562067691 -0.038116320731449584 4.2272798056538269e-07];  % mm
  | smiData.Solid(17).MoI = [220.69606748985959 143.16584265871566 142.83835130647245];  % kg*mm^2
  | smiData.Solid(17).PoI = [-0.14978797789806547 1.4186799978182654e-06 0.070880231556233561];  % kg*mm^2
  | smiData.Solid(17).color = [0.50196078431372548 0.50196078431372548 0.50196078431372548];
  | smiData.Solid(17).opacity = 1;
  | smiData.Solid(17).ID = 'limiteur couple*:*Defaut';
  | 
  | %Inertia Type - Custom
  | %Visual Properties - Simple
  | smiData.Solid(18).mass = 0.0011210856237282797;  % kg
  | smiData.Solid(18).CoM = [0 -0.1681226089471074 22.500000000000004];  % mm
  | smiData.Solid(18).MoI = [0.19316156497796899 0.1937607518512055 0.010617336392666694];  % kg*mm^2
  | smiData.Solid(18).PoI = [0 0 0];  % kg*mm^2
  | smiData.Solid(18).color = [0.50196078431372548 1 0];
  | smiData.Solid(18).opacity = 1;
  | smiData.Solid(18).ID = 'mecanindus*:*Defaut';
  | 
  | %Inertia Type - Custom
  | %Visual Properties - Simple
  | smiData.Solid(19).mass = 0.003126667885608054;  % kg
  | smiData.Solid(19).CoM = [-0.99999999999998745 87.5 0];  % mm
  | smiData.Solid(19).MoI = [0.44924188257307629 0.26644360703666331 0.2664436070366632];  % kg*mm^2
  | smiData.Solid(19).PoI = [0 0 0];  % kg*mm^2
  | smiData.Solid(19).color = [0.75294117647058822 0.75294117647058822 0.75294117647058822];
  | smiData.Solid(19).opacity = 1;
  | smiData.Solid(19).ID = 'BI 6004*:*Defaut';
  | 
  | %Inertia Type - Custom
  | %Visual Properties - Simple
  | smiData.Solid(20).mass = 0.00011309733552923285;  % kg
  | smiData.Solid(20).CoM = [-0.99999999999999312 103.00000000000001 0];  % mm
  | smiData.Solid(20).MoI = [0.0004071504079052391 0.0004071504079052391 0.0004071504079052391];  % kg*mm^2
  | smiData.Solid(20).PoI = [0 0 0];  % kg*mm^2
  | smiData.Solid(20).color = [0.75294117647058822 0.75294117647058822 0.75294117647058822];
  | smiData.Solid(20).opacity = 1;
  | smiData.Solid(20).ID = 'bille 6004*:*Defaut';
  | 
  | %Inertia Type - Custom
  | %Visual Properties - Simple
  | smiData.Solid(21).mass = 0.005062440714193206;  % kg
  | smiData.Solid(21).CoM = [-0.99999999999999478 87.499999999999986 0];  % mm
  | smiData.Solid(21).MoI = [1.8772337333916647 1.0046255872291054 1.004625587229105];  % kg*mm^2
  | smiData.Solid(21).PoI = [0 0 0];  % kg*mm^2
  | smiData.Solid(21).color = [0.75294117647058822 0.75294117647058822 0.75294117647058822];
  | smiData.Solid(21).opacity = 1;
  | smiData.Solid(21).ID = 'BE 6004*:*Defaut';
  | 
  | %Inertia Type - Custom
  | %Visual Properties - Simple
  | smiData.Solid(22).mass = 0.0020327413465664949;  % kg
  | smiData.Solid(22).CoM = [9.2223501191319457 0 0];  % mm
  | smiData.Solid(22).MoI = [0.037805543111694873 0.14489477777499224 0.14489477777499221];  % kg*mm^2
  | smiData.Solid(22).PoI = [0 0 0];  % kg*mm^2
  | smiData.Solid(22).color = [0 0.50196078431372548 1];
  | smiData.Solid(22).opacity = 1;
  | smiData.Solid(22).ID = 'doigt*:*Defaut';
  | 
  | %Inertia Type - Custom
  | %Visual Properties - Simple
  | smiData.Solid(23).mass = 0.082681748252273812;  % kg
  | smiData.Solid(23).CoM = [63.153946673579597 1.1527048820682519e-06 -0.15456952451571168];  % mm
  | smiData.Solid(23).MoI = [11.518281720972663 293.97325795091268 293.87206081952456];  % kg*mm^2
  | smiData.Solid(23).PoI = [2.9340495108749846e-06 -0.69208028028111179 -8.3838155325792233e-06];  % kg*mm^2
  | smiData.Solid(23).color = [1 0.50196078431372548 0.50196078431372548];
  | smiData.Solid(23).opacity = 1;
  | smiData.Solid(23).ID = 'axe de sortie*:*Defaut';
  | 
  | %Inertia Type - Custom
  | %Visual Properties - Simple
  | smiData.Solid(24).mass = 0.27193713488245563;  % kg
  | smiData.Solid(24).CoM = [10.720533876975381 0.13871068217264801 7.8965473223586728e-05];  % mm
  | smiData.Solid(24).MoI = [911.69992496943655 476.03963844096091 474.14945060235669];  % kg*mm^2
  | smiData.Solid(24).PoI = [3.0513592674507086e-06 0.00011210388872882407 0.12152337071135293];  % kg*mm^2
  | smiData.Solid(24).color = [0.75294117647058822 0.75294117647058822 0.75294117647058822];
  | smiData.Solid(24).opacity = 1;
  | smiData.Solid(24).ID = 'croix*:*Defaut';
  | 
  | %Inertia Type - Custom
  | %Visual Properties - Simple
  | smiData.Solid(25).mass = 0.012500133342040136;  % kg
  | smiData.Solid(25).CoM = [22.875708221300044 0 6.0000000000000009];  % mm
  | smiData.Solid(25).MoI = [1.5119394555587713 3.3296132639442688 4.541549519294076];  % kg*mm^2
  | smiData.Solid(25).PoI = [0 0 0];  % kg*mm^2
  | smiData.Solid(25).color = [0 1 0];
  | smiData.Solid(25).opacity = 1;
  | smiData.Solid(25).ID = 'capteur*:*Defaut';
  | 
  | %Inertia Type - Custom
  | %Visual Properties - Simple
  | smiData.Solid(26).mass = 0.0011173912024876611;  % kg
  | smiData.Solid(26).CoM = [0 0 18.182336055242565];  % mm
  | smiData.Solid(26).MoI = [0.10289928272414046 0.10289928272414046 0.0088659711058604561];  % kg*mm^2
  | smiData.Solid(26).PoI = [0 0 0];  % kg*mm^2
  | smiData.Solid(26).color = [0.50196078431372548 1 1];
  | smiData.Solid(26).opacity = 1;
  | smiData.Solid(26).ID = 'vis M6x25*:*Defaut';
  | 
  | %Inertia Type - Custom
  | %Visual Properties - Simple
  | smiData.Solid(27).mass = 0.0018838686010957345;  % kg
  | smiData.Solid(27).CoM = [0 -5.4999999999999991 -0.13414733414733332];  % mm
  | smiData.Solid(27).MoI = [0.073245885891853116 0.11568316608532395 0.073245885891853102];  % kg*mm^2
  | smiData.Solid(27).PoI = [0 0 0];  % kg*mm^2
  | smiData.Solid(27).color = [0 0 1];
  | smiData.Solid(27).opacity = 1;
  | smiData.Solid(27).ID = 'rouleau galet*:*Defaut';
  | 
  | %Inertia Type - Custom
  | %Visual Properties - Simple
  | smiData.Solid(28).mass = 0.18246752943347352;  % kg
  | smiData.Solid(28).CoM = [24.534251621189323 -5.7879669054264076 0];  % mm
  | smiData.Solid(28).MoI = [263.57971176382989 182.19471790534803 128.43301076436617];  % kg*mm^2
  | smiData.Solid(28).PoI = [-0.45128978468816133 0 -4.2606377726098943];  % kg*mm^2
  | smiData.Solid(28).color = [0.792156862745098 0.81960784313725488 0.93333333333333335];
  | smiData.Solid(28).opacity = 1;
  | smiData.Solid(28).ID = 'indexeur*:*Defaut';
  | 
  | %Inertia Type - Custom
  | %Visual Properties - Simple
  | smiData.Solid(29).mass = 0.00070510652087749906;  % kg
  | smiData.Solid(29).CoM = [-1.216054972847654e-07 0.00032694383918773092 3.2500025620456685];  % mm
  | smiData.Solid(29).MoI = [0.01260539418276062 0.012605461767665449 0.020330696114904963];  % kg*mm^2
  | smiData.Solid(29).PoI = [-1.0148091697554322e-08 2.0074966733223823e-09 -1.0758911587445887e-09];  % kg*mm^2
  | smiData.Solid(29).color = [0.792156862745098 0.81960784313725488 0.93333333333333335];
  | smiData.Solid(29).opacity = 1;
  | smiData.Solid(29).ID = 'ecrou M8*:*Defaut';
  | 
  | %Inertia Type - Custom
  | %Visual Properties - Simple
  | smiData.Solid(30).mass = 0.08729961170300711;  % kg
  | smiData.Solid(30).CoM = [54.754906437773954 -0.26369586050273175 1.1459860194635749e-06];  % mm
  | smiData.Solid(30).MoI = [13.168045483824388 210.49722743800717 210.55321190117937];  % kg*mm^2
  | smiData.Solid(30).PoI = [-7.0726095582996631e-07 -7.6923541852263123e-06 -0.0070983165488733083];  % kg*mm^2
  | smiData.Solid(30).color = [0.792156862745098 0.81960784313725488 0.93333333333333335];
  | smiData.Solid(30).opacity = 1;
  | smiData.Solid(30).ID = 'arbre moteur*:*Defaut';
  | 
  | %Inertia Type - Custom
  | %Visual Properties - Simple
  | smiData.Solid(31).mass = 0.0021915226752666802;  % kg
  | smiData.Solid(31).CoM = [0 0 13.999999999999998];  % mm
  | smiData.Solid(31).MoI = [0.1558784807258054 0.1558784807258054 0.027311259019396104];  % kg*mm^2
  | smiData.Solid(31).PoI = [0 0 0];  % kg*mm^2
  | smiData.Solid(31).color = [0.75294117647058822 0.75294117647058822 0.75294117647058822];
  | smiData.Solid(31).opacity = 1;
  | smiData.Solid(31).ID = 'goupille D10*:*Defaut';
  | 
  | %Inertia Type - Custom
  | %Visual Properties - Simple
  | smiData.Solid(32).mass = 0.046586902287852075;  % kg
  | smiData.Solid(32).CoM = [50.128123256344736 35 5.9530004291266971];  % mm
  | smiData.Solid(32).MoI = [18.510271234791187 80.02940297276696 97.421794369825591];  % kg*mm^2
  | smiData.Solid(32).PoI = [0 -0.033124000360619944 1.0484364277875708];  % kg*mm^2
  | smiData.Solid(32).color = [0.792156862745098 0.81960784313725488 0.93333333333333335];
  | smiData.Solid(32).opacity = 1;
  | smiData.Solid(32).ID = 'maneton*:*Defaut';
  | 
  | %Inertia Type - Custom
  | %Visual Properties - Simple
  | smiData.Solid(33).mass = 0.00020734511513692614;  % kg
  | smiData.Solid(33).CoM = [1.0000000000000102 0 0];  % mm
  | smiData.Solid(33).MoI = [0.0067387162419500612 0.0034384731593540001 0.0034384731593540001];  % kg*mm^2
  | smiData.Solid(33).PoI = [0 0 0];  % kg*mm^2
  | smiData.Solid(33).color = [0.792156862745098 0.81960784313725488 0.93333333333333335];
  | smiData.Solid(33).opacity = 1;
  | smiData.Solid(33).ID = 'rondelle galet*:*Defaut';
  | 
  | %Inertia Type - Custom
  | %Visual Properties - Simple
  | smiData.Solid(34).mass = 0.0021222149525382825;  % kg
  | smiData.Solid(34).CoM = [14.173587536749354 0 0];  % mm
  | smiData.Solid(34).MoI = [0.024769763580159542 0.23967590250872042 0.23967590250872042];  % kg*mm^2
  | smiData.Solid(34).PoI = [0 0 0];  % kg*mm^2
  | smiData.Solid(34).color = [0.792156862745098 0.81960784313725488 0.93333333333333335];
  | smiData.Solid(34).opacity = 1;
  | smiData.Solid(34).ID = 'axe galet*:*Defaut';
  | 
  | %Inertia Type - Custom
  | %Visual Properties - Simple
  | smiData.Solid(35).mass = 0.0021136460032938485;  % kg
  | smiData.Solid(35).CoM = [2.9999999999999996 2.9999999999999996 30.000000000000004];  % mm
  | smiData.Solid(35).MoI = [0.6144505779185081 0.61432334341603778 0.012554641517292707];  % kg*mm^2
  | smiData.Solid(35).PoI = [0 0 0];  % kg*mm^2
  | smiData.Solid(35).color = [0.792156862745098 0.81960784313725488 0.93333333333333335];
  | smiData.Solid(35).opacity = 1;
  | smiData.Solid(35).ID = 'clavette*:*Defaut';
  | 
  | %Inertia Type - Custom
  | %Visual Properties - Simple
  | smiData.Solid(36).mass = 0.0026734953482049142;  % kg
  | smiData.Solid(36).CoM = [2.0000000000001075 0.49999999999999917 0];  % mm
  | smiData.Solid(36).MoI = [0.31714338568080791 0.16213635330467738 0.16213635330467741];  % kg*mm^2
  | smiData.Solid(36).PoI = [0 0 0];  % kg*mm^2
  | smiData.Solid(36).color = [0.792156862745098 0.81960784313725488 0.93333333333333335];
  | smiData.Solid(36).opacity = 1;
  | smiData.Solid(36).ID = 'rondelle arbre moteur*:*Defaut';
  | 
  | %Inertia Type - Custom
  | %Visual Properties - Simple
  | smiData.Solid(37).mass = 0.00083464786366457984;  % kg
  | smiData.Solid(37).CoM = [0 0 12.621291599341518];  % mm
  | smiData.Solid(37).MoI = [0.034906470394779149 0.034906470394779149 0.0075936260811565928];  % kg*mm^2
  | smiData.Solid(37).PoI = [0 0 0];  % kg*mm^2
  | smiData.Solid(37).color = [0.792156862745098 0.81960784313725488 0.93333333333333335];
  | smiData.Solid(37).opacity = 1;
  | smiData.Solid(37).ID = 'vis M6x15*:*Defaut';
  | 
  | 
  | %============= Joint =============%
  | %X Revolute Primitive (Rx) %Y Revolute Primitive (Ry) %Z Revolute Primitive (Rz)
  | %X Prismatic Primitive (Px) %Y Prismatic Primitive (Py) %Z Prismatic Primitive (Pz) %Spherical Primitive (S)
  | %Constant Velocity Primitive (CV) %Lead Screw Primitive (LS)
  | %Position Target (Pos)
  | 
  | %Initialize the RevoluteJoint structure array by filling in null values.
  | smiData.RevoluteJoint(3).Rz.Pos = 0.0;
  | smiData.RevoluteJoint(3).ID = '';
  | 
  | smiData.RevoluteJoint(1).Rz.Pos = -1.0548706503622822e-14;  % deg
  | smiData.RevoluteJoint(1).ID = '[Bati-1:-:Croix_de_Malte-1]';
  | 
  | smiData.RevoluteJoint(2).Rz.Pos = -44.64966140570008;  % deg
  | smiData.RevoluteJoint(2).ID = '[Bati-1:-:Moteur-1]';
  | 
  | %This joint has been chosen as a cut joint. Simscape Multibody treats cut joints as algebraic constraints to solve closed kinematic loops. The imported model does not use the state target data for this joint.
  | smiData.RevoluteJoint(3).Rz.Pos = 45.810842911106427;  % deg
  | smiData.RevoluteJoint(3).ID = '[rouleau galet-1:-:Moteur-1]';
undefined symbols (not defined in the file or in its folder): smiData, X, Y, Z
libraries: sm_lib x218, nesl_utility x4
(part 1 of 5)
settings Model: Creator=Renaud  LastModifiedBy=Renaud

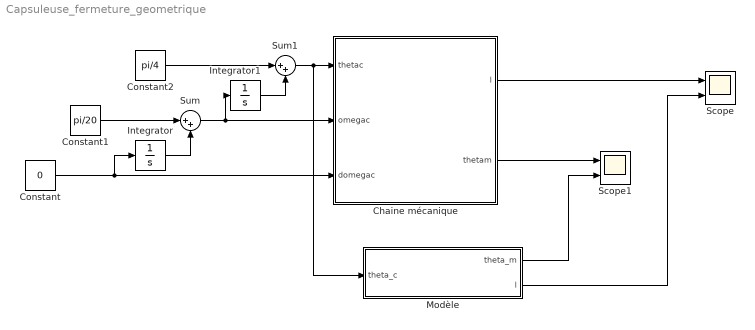
== system Capsuleuse_fermeture_geometrique ==
  Chaine mécanique : Subsystem
      mask Display: image('$imagefile'); % Use "Edit Image" on toolstrip to change.
  Constant : Constant  Value=0
  Constant1 : Constant  Value=pi/20
  Constant2 : Constant  Value=pi/4
  Integrator : Integrator
  Integrator1 : Integrator
  Modèle : MATLAB Function  TreatAsAtomicUnit=on
  Scope : Scope  NumInputPorts=2
  Scope1 : Scope  NumInputPorts=2
  Sum : Sum  Inputs=|++
  Sum1 : Sum  Inputs=|++
  wires:
  Chaine mécanique/1(l) -> Scope/1
  Chaine mécanique/2(thetam) -> Scope1/1
  Constant2/1 -> Sum1/1
  Sum1/1 -> Modèle/1(theta_c), Chaine mécanique/1(thetac)
  Constant/1 -> Integrator/1, Chaine mécanique/3(domegac)
  Constant1/1 -> Sum/1
  Integrator1/1 -> Sum1/2
  Sum/1 -> Chaine mécanique/2(omegac), Integrator1/1
  Integrator/1 -> Sum/2
  Modèle/1(theta_m) -> Scope1/2
  Modèle/2(l) -> Scope/2
